simulink model "TruckBenchmark"  (R2023a)
settings: Solver=FixedStepAuto  StartTime=0.0  StopTime=sim_time  FixedStep=control.Ts  MaxStep=1  RelTol=1e-3  EnableMultiTasking=on
StartFcn:
  | tic
StopFcn:
  | simt=toc;
  | fprintf('Simulation time %.3f s\n',simt)
  | TruckBenchmark_Evaluation
values from neighbouring files (symbols this model uses):
  attack_duration = input('Enter the duration of each attack: ')    [RunMe.m]
  attack_freq = input('Enter the desired frequency of attack: ')    [RunMe.m]
  attack_time = input('Enter the time for attack: ')    [RunMe.m]
  attack_type = input('Select the type of Attack (1= Fuzzy, 2=spoofing, 3=Plateau, 4=Replay Attack, 5 = GAttack, 6= C-GAttack, 7= No Attack, 8 = Denial of Service):')    [RunMe.m]
  can_sample_time = 0.001    [runSim.m]
  clutch_pos = TruckBenchmark_Result.find('clutch_pos').Values    [TruckBenchmark_Evaluation.m]
  control =     [TruckBenchmark_Control.mat]
  cruise_profile = input('Select Cruise Profile (Step decrease = 1, Constant 80kph = 2): ')    [RunMe.m]
  curr_gear = TruckBenchmark_Result.find('curr_gear').Values    [TruckBenchmark_Evaluation.m]
  DoS = 0    [RunMe.m]
  gattack_data = interp1(original_time, data, desired_time, 'linear')    [RunMe.m]
  gattack_time = desired_time    [RunMe.m]
  k_slope = TruckBenchmark_Result.find('k_slope').Values    [TruckBenchmark_Evaluation.m]
  lambda = TruckBenchmark_Result.find('lambda').Values    [TruckBenchmark_Evaluation.m]
  model =     [TruckBenchmark_Data.mat]
  n_engine = TruckBenchmark_Result.find('n_engine').Values    [TruckBenchmark_Evaluation.m]
  road = scenario.road    [runSim.m]
  scenario =     [Sodertalje_Norrkoping_Scenario.mat]
  sim_time = input('Enter the total simulation time: ')    [RunMe.m]
  spoofed_value = input('Set the spoofing value:')    [RunMe.m]
  ts = struct('orig_30kph', ts_orig_30kph, 'gen_30kph', ts_gen_30kph, 'orig_40kph', ts_orig_40kph, 'gen_40kph', ts_gen_40kph, 'orig_50kph', ts_orig_50kph, 'gen_50kph', ts_gen_50kph, 'orig_60kph', ts_orig_60kph, 'gen_60kph', ts_gen_60kph,'orig_70kph', ts_orig_70kph, 'gen_70kph', ts_gen_70kph, 'orig_80kph', ts_orig_80kph, 'gen_80kph', ts_gen_80kph, 'orig_90kph', ts_orig_90kph, 'gen_90kph', ts_gen_90kph)    [data_to_mat.m]
  v_vehicle = 0    [RunMe.m]    (also in TruckBenchmark_Evaluation.m = TruckBenchmark_Result.find('v_vehicle').Values)
undefined symbols (not defined in the file or in its folder): canChannel, CCVS, DiscIntNeverNeededParam, dm_airInlet, EGF1, ESSI, ETC2, gcbh, IMT1, n_t, p_inletManifold, r_egr, VD, VDHR, x_distance
libraries: j1939protocollib x25, simulink x5, canlib x2, j1939tllib x2, canmsglib x1, vntj1939tllib x1, slpidlib x1
(part 2 of 4)

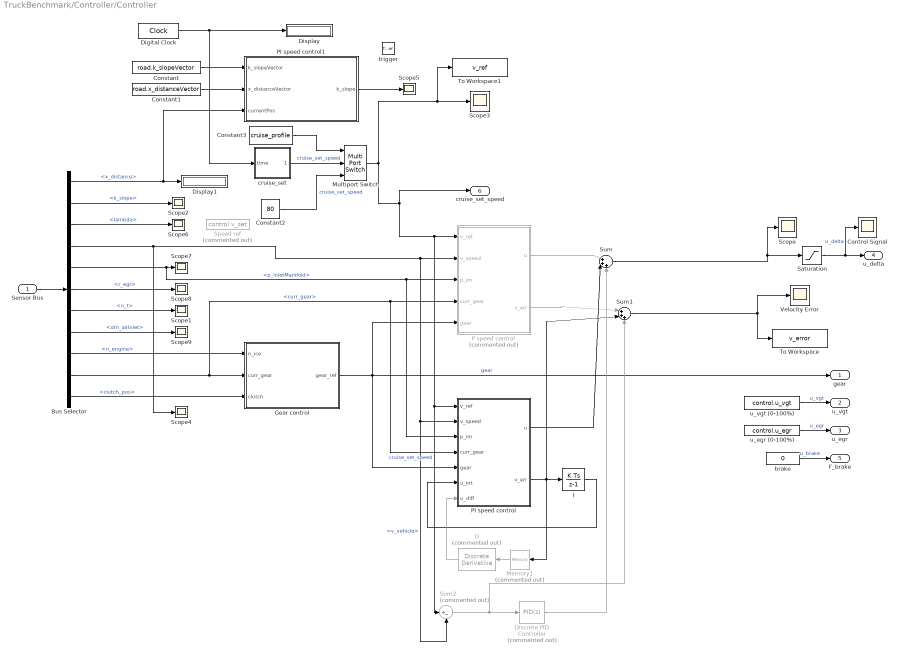
== system TruckBenchmark/Controller/Controller ==
  Sensor Bus : Inport
  trigger : TriggerPort  TriggerType=function-call  VariantControl=(inherit)  PortDimensions=1
  Bus Selector : BusSelector  OutputSignals=x_distance,k_slope,lambda,v_vehicle,p_inletManifold,r_egr,n_t,dm_airInlet,n_engine,curr_gear,clutch_pos
  Constant : Constant  Value=road.k_slopeVector
  Constant1 : Constant  Value=road.x_distanceVector
  Constant2 : Constant  Value=80
  Constant3 : Constant  Value=cruise_profile
  Control Signal : Scope
  D : simulink/Discrete/Discrete Derivative  Commented=on  gainval=1.0  ICPrevScaledInput=0.0  OutMin=[]  OutMax=[]  OutDataType=fixdt(1, 16)  OutScaling=2^-10  DoSatur=off
  Digital Clock : DigitalClock  SampleTime=-1
  Discrete PID Controller : slpidlib/PID Controller  Commented=on  Controller=PID  Form=Parallel  TimeDomain=Discrete-time  UseExternalTs=off  SampleTime=-1  IntegratorMethod=Forward Euler  FilterMethod=Forward Euler  ControllerParametersSource=internal  P=300  I=150  UseKiTs=off  D=0  N=1  UseFilter=on  TunerSelectOption=Transfer Function Based (PID Tuner App)  InitialConditionSource=internal  InitialConditionForIntegrator=0  InitialConditionForFilter=0  DifferentiatorICPrevScaledInput=0  ExternalReset=none  TrackingMode=off  Kt=1  LimitOutput=off  SatLimitsSource=internal  UpperSaturationLimit=inf  LowerSaturationLimit=-inf  LinearizeAsGain=off  AntiWindupMode=none  Kb=1  LimitIntegrator=off  UpperIntegratorSaturationLimit=inf  LowerIntegratorSaturationLimit=-inf  POutMin=[]  POutMax=[]  IOutMin=[]  IOutMax=[]  DOutMin=[]  DOutMax=[]  NOutMin=[]  NOutMax=[]  SumOutMin=[]  SumOutMax=[]  SaturationOutMin=[]  SaturationOutMax=[]  PParamMin=[]  PParamMax=[]  IParamMin=[]  IParamMax=[]  DParamMin=[]  DParamMax=[]  NParamMin=[]  NParamMax=[]  KbParamMin=[]  KbParamMax=[]  KtParamMin=[]  KtParamMax=[]  KbOutMin=[]  KbOutMax=[]  KtOutMin=[]  KtOutMax=[]  IntegratorOutMin=[]  IntegratorOutMax=[]  FilterOutMin=[]  FilterOutMax=[]  SumI1OutMin=[]  SumI1OutMax=[]  SumI2OutMin=[]  SumI2OutMax=[]  SumI3OutMin=[]  SumI3OutMax=[]  SumI4OutMin=[]  SumI4OutMax=[]  SumDOutMin=[]  SumDOutMax=[]  DifferentiatorOutMin=[]  DifferentiatorOutMax=[]  FilterDiffOutCoefMin=[]  FilterDiffOutCoefMax=[]  ReciprocalOutMin=[]  ReciprocalOutMax=[]  SumDenOutMin=[]  SumDenOutMax=[]  SumNumOutMin=[]  SumNumOutMax=[]  DivideOutMin=[]  DivideOutMax=[]  UdiffTsProdOutMin=[]  UdiffTsProdOutMax=[]  NTsProdOutMin=[]  NTsProdOutMax=[]  UintegralTsProdOutMin=[]  UintegralTsProdOutMax=[]  UngainTsProdOutMin=[]  UngainTsProdOutMax=[]  ClampingZeroOutDataTypeStr=Inherit: Inherit via back propagation  ClampingZeroOutMin=[]  ClampingZeroOutMax=[]  FilterDenConstantOutDataTypeStr=Inherit: Inherit via back propagation  FilterDenConstantOutMin=[]  FilterDenConstantOutMax=[]  PCopyOutDataTypeStr=Inherit: Inherit via back propagation  PCopyOutMin=[]  PCopyOutMax=[]  NCopyOutDataTypeStr=Inherit: Inherit via back propagation  NCopyOutMin=[]  NCopyOutMax=[]  IntegratorContinuousStateAttributes=''  IntegratorStateMustResolveToSignalObject=off  IntegratorRTWStateStorageClass=Auto  FilterContinuousStateAttributes=''  FilterStateMustResolveToSignalObject=off  FilterRTWStateStorageClass=Auto  ParallelPVariant=InternalParameters  IdealPVariant=Disabled  IVariant=InternalParameters  DVariant=InternalParameters  IntegratorVariant=Discrete  SatVariant=Disabled  AWVariant=Passthrough  PCopyVariant=Disabled  TRVariant=Disabled  FdbkBlocksVariant=Forward  IdealPFdbkVariant=Disabled  SatFdbkVariant=Disabled  DerivativeFilterVariant=ForwardEulerFilter  NVariant=InternalParameters  NCopyVariant=Disabled  FilterICVariant=InternalICsFilter  IntegratorICVariant=InternalICs  ExternalResetVariant=Disabled  TRSumVariant=Passthrough  SumFdbkVariant=Disabled  SumVariant=Sum_PID  TsampFilterVariant=InternalTs  TsampNgainVariant=Passthrough  TsampIntegralVariant=Disabled_SignalSpec  ExternalSaturationOutDataTypeStr=Inherit: Same as second input
      settings: LibrarySourceBlock=simulink/Discrete/Discrete PID Controller
  Display : Display
  Display1 : Display
  Gear control : MATLAB Function  TreatAsAtomicUnit=on
  I : DiscreteIntegrator  SampleTime=-1  ICPrevOutput=DiscIntNeverNeededParam  ICPrevScaledInput=DiscIntNeverNeededParam
  Memory1 : Memory  Commented=on  InitialCondition=40  InheritSampleTime=on
  Multiport Switch : MultiPortSwitch  Inputs=2  SaturateOnIntegerOverflow=off  InputSameDT=off
  P speed control : MATLAB Function  Commented=on  TreatAsAtomicUnit=on
  PI speed control : MATLAB Function  TreatAsAtomicUnit=on
  PI speed control1 : MATLAB Function  TreatAsAtomicUnit=on
  Saturation : Saturate  UpperLimit=300  LowerLimit=0
  Scope{,1..9} (10 alike) : Scope
  Speed ref : Constant  Commented=on  Value=control.v_set
  Sum : Sum  Inputs=|+++
  Sum1 : Sum  Inputs=|+++
  Sum2 : Sum  Commented=on  Inputs=|+-
  To Workspace : ToWorkspace  VariableName=v_error  SampleTime=-1
  To Workspace1 : ToWorkspace  VariableName=v_ref  SaveFormat=Timeseries  SampleTime=-1
  Velocity Error : Scope
  brake : Constant  Value=0
  cruise_set : MATLAB Function  TreatAsAtomicUnit=on
  u_egr (0-100%) : Constant  Value=control.u_egr
  u_vgt (0-100%) : Constant  Value=control.u_vgt
  gear : Outport  InitialOutput=0
  u_vgt : Outport  Port=2  InitialOutput=0
  u_egr : Outport  Port=3  InitialOutput=0
  u_delta : Outport  Port=4  InitialOutput=0
  F_brake : Outport  Port=5  InitialOutput=0
  cruise_set_speed : Outport  Port=6  InitialOutput=0
  wires:
  Saturation/1 -> Control Signal/1, u_delta/1  "u_delta"
  u_vgt (0-100%)/1 -> u_vgt/1  "u_vgt"
  u_egr (0-100%)/1 -> u_egr/1  "u_egr"
  brake/1 -> F_brake/1  "u_brake"
  Digital Clock/1 -> cruise_set/1(time), Display/1
  Constant/1 -> PI speed control1/1(k_slopeVector)
  Constant1/1 -> PI speed control1/2(x_distanceVector)
  PI speed control1/1(k_slope) -> Scope5/1
  Sensor Bus/1 -> Bus Selector/1
  Bus Selector/5 -> Scope7/1, PI speed control/3(p_im), P speed control/3(p_im)  "<p_inletManifold>"
  Bus Selector/3 -> Scope6/1  "<lambda>"
  Bus Selector/1 -> Display1/1, PI speed control1/3(currentPos)  "<x_distance>"
  Bus Selector/6 -> Scope8/1  "<r_egr>"
  Bus Selector/2 -> Scope2/1  "<k_slope>"
  Bus Selector/8 -> Scope9/1  "<dm_airInlet>"
  Bus Selector/9 -> Gear control/1(n_ice)  "<n_engine>"
  Bus Selector/4 -> Scope4/1, Sum2/2, PI speed control/2(v_speed), P speed control/2(v_speed)  "<v_vehicle>"
  Bus Selector/7 -> Scope1/1  "<n_t>"
  Bus Selector/10 -> Gear control/2(curr_gear), PI speed control/4(curr_gear), P speed control/4(curr_gear)  "<curr_gear>"
  Gear control/1(gear_ref) -> PI speed control/5(gear), gear/1, P speed control/5(gear)  "gear"
  Bus Selector/11 -> Gear control/3(clutch)  "<clutch_pos>"
  Sum1/1 -> To Workspace/1, Velocity Error/1
  Multiport Switch/1 -> cruise_set_speed/1, P speed control/1(v_ref), PI speed control/1(v_ref), Sum2/1, Scope3/1, To Workspace1/1  "cruise_set_speed"
  Sum/1 -> Saturation/1, Scope/1
  P speed control/1(u) -> Sum/1
  PI speed control/1(u) -> Sum/2
  P speed control/2(v_err) -> Sum1/1
  PI speed control/2(v_err) -> I/1, Memory1/1, Sum1/2
  I/1 -> PI speed control/6(u_int)
  Sum2/1 -> Sum1/3, Discrete PID Controller/1
  Discrete PID Controller/1 -> Sum/3
  D/1 -> PI speed control/7(u_diff)
  Memory1/1 -> D/1
  cruise_set/1(cruise_set_speed) -> Multiport Switch/2  "cruise_set_speed"
  Constant2/1 -> Multiport Switch/3  "cruise_set_speed"
  Constant3/1 -> Multiport Switch/1

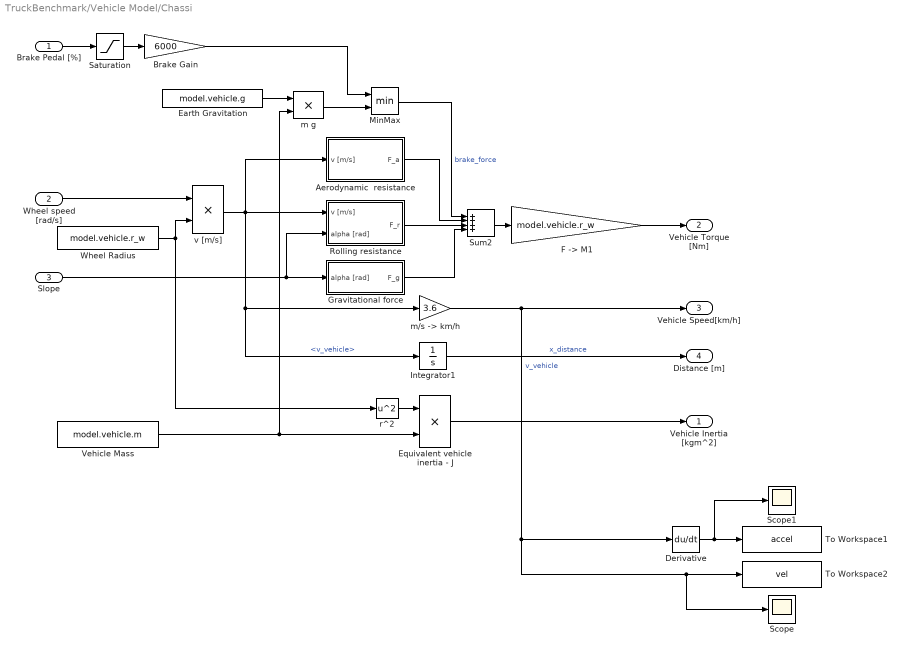
== system TruckBenchmark/Vehicle Model/Chassi ==
  Brake Pedal [%] : Inport
  Wheel speed [rad/s] : Inport  Port=2
  Slope : Inport  Port=3
  Aerodynamic  resistance : Subsystem  mask(Air Drag Subsystem){C_d=model.vehicle.C_d, rho=model.vehicle.rho, Area=model.vehicle.A}
      mask prompts: C_d "C_d - Drag Coefficient  [-]"; rho "rho - Air density [kg/m^3]"; Area "A - Area [m^2]"
      mask help:
      | Calculates the air drag given input vehicle velocity, v, constant values on
      | cross section area, A, drag coefficient, C_d, and air density, rho.
      |
      | Implemented Equation:
      | F_a=0.5 rho C_d A v^2
  Brake Gain : Gain  Gain=6000  SaturateOnIntegerOverflow=on  OutDataTypeStr=Inherit: Same as input  ParamDataTypeStr=Inherit: Same as input
  Derivative : Derivative
  Earth Gravitation : Constant  Value=model.vehicle.g
  Equivalent vehicle inertia - J : Product  SaturateOnIntegerOverflow=on  OutDataTypeStr=Inherit: Same as first input
  "F -> M1" : Gain  Gain=model.vehicle.r_w  SaturateOnIntegerOverflow=on  OutDataTypeStr=Inherit: Same as input  ParamDataTypeStr=Inherit: Same as input
  Gravitational force : Subsystem  mask(Rolling resistance subsystem){m=model.vehicle.m, g=model.vehicle.g}
      mask prompts: m "m - Vehicle mass"; g "g - Gravity of Earth"
      mask help:
      | Calculates the gravitational force given the road slope, alpha, as input
      | and constants for vehicle mass, m, and earth gravitation.
      |
      | Model Equation:
      | F_r = m g sin(alpha)
  Integrator1 : Integrator  LimitOutput=on  LowerSaturationLimit=0
  MinMax : MinMax  Inputs=2
  Rolling resistance : Subsystem  mask(Rolling resistance subsystem){m=model.vehicle.m, g=model.vehicle.g, c_r0=model.vehicle.c_r0, c_r1=model.vehicle.c_r1}
      mask prompts: m "m - Vehicle massm"; g "g - Gravity of Earth"; c_r0 "c_r0 - Rolling resistance coeff"; c_r1 "c_r1 - Rolling resistanc coeff"
      mask help:
      | Calculates the rolling resistance force of a vehicle of mass, m, at
      | vehicle speed, v.
      |
      | Model Equation:
      | F_r = m g cos(alpha) (c_r0 + c_r1 v)
  Saturation : Saturate  UpperLimit=100  LowerLimit=0
  Scope : Scope
  Scope1 : Scope
  Sum2 : Sum  Inputs=++++  SaturateOnIntegerOverflow=on
  To Workspace1 : ToWorkspace  VariableName=accel  SampleTime=-1
  To Workspace2 : ToWorkspace  VariableName=vel  SampleTime=-1
  Vehicle Mass : Constant  Value=model.vehicle.m
  Wheel Radius : Constant  Value=model.vehicle.r_w
  m g : Product  SaturateOnIntegerOverflow=on  OutDataTypeStr=Inherit: Same as first input
  "m/s -> km/h" : Gain  Gain=3.6  SaturateOnIntegerOverflow=on  OutDataTypeStr=Inherit: Same as input  ParamDataTypeStr=Inherit: Same as input
  r^2 : Math  Operator=square  SignedPower=on
  v [m/s] : Product  SaturateOnIntegerOverflow=on  OutDataTypeStr=Inherit: Same as first input
  Vehicle Inertia [kgm^2] : Outport  VectorParamsAs1DForOutWhenUnconnected=off
  Vehicle Torque [Nm] : Outport  Port=2  VectorParamsAs1DForOutWhenUnconnected=off
  Vehicle Speed[km/h] : Outport  Port=3  VectorParamsAs1DForOutWhenUnconnected=off
  Distance [m] : Outport  Port=4  VectorParamsAs1DForOutWhenUnconnected=off
  wires:
  Brake Pedal [%]/1 -> Saturation/1
  Wheel Radius/1 -> r^2/1, v [m/s]/2
  "m/s -> km/h"/1 -> Scope/1, To Workspace2/1, Derivative/1, Vehicle Speed[km/h]/1  "v_vehicle"
  "F -> M1"/1 -> Vehicle Torque [Nm]/1
  Equivalent vehicle inertia - J/1 -> Vehicle Inertia [kgm^2]/1
  Wheel speed [rad/s]/1 -> v [m/s]/1
  Sum2/1 -> "F -> M1"/1
  Slope/1 -> Rolling resistance/2(alpha [rad]), Gravitational force/1(alpha [rad])
  r^2/1 -> Equivalent vehicle inertia - J/1
  Vehicle Mass/1 -> m g/2, Equivalent vehicle inertia - J/2
  Integrator1/1 -> Distance [m]/1  "x_distance"
  Brake Gain/1 -> MinMax/1
  m g/1 -> MinMax/2
  Earth Gravitation/1 -> m g/1
  Saturation/1 -> Brake Gain/1
  MinMax/1 -> Sum2/1  "brake_force"
  Aerodynamic  resistance/1(F_a) -> Sum2/2
  Rolling resistance/1(F_r) -> Sum2/3
  Gravitational force/1(F_g) -> Sum2/4
  v [m/s]/1 -> Aerodynamic  resistance/1(v [m/s]), Rolling resistance/1(v [m/s]), Integrator1/1, "m/s -> km/h"/1  "<v_vehicle>"
  Derivative/1 -> Scope1/1, To Workspace1/1

== system TruckBenchmark/Vehicle Model/Clutch and Transmission ==
  M_e [Nm] : Inport
  Gear : Inport  Port=2
  Clutch Pos [0...1] : Inport  Port=3
  J_e : Inport  Port=4
  M_veh [Nm] : Inport  Port=5
  J_veh : Inport  Port=6
  Clutch Transfer : Subsystem
  Engine Dynamics : Subsystem
  Final Drive gear ratio : Gain  Gain=model.transmission.i_f
  Gear box gear ratios : Lookup  InputValues=model.transmission.r_gearNumbers  Table=model.transmission.r_gearRatios
  Mux : Mux  Inputs=5
  Speed Difference Clutch Limits : Subsystem
  Vehicle Dynamics : Subsystem
  w_e [rad/s] : Outport  VectorParamsAs1DForOutWhenUnconnected=off
  w_wheel [rad/s] : Outport  Port=2  VectorParamsAs1DForOutWhenUnconnected=off
  wires:
  M_e [Nm]/1 -> Engine Dynamics/2(Tq_e), Mux/1
  J_e/1 -> Engine Dynamics/3(J_e), Mux/2
  Gear/1 -> Gear box gear ratios/1
  M_veh [Nm]/1 -> Vehicle Dynamics/2(Tq_veh), Mux/3
  J_veh/1 -> Vehicle Dynamics/3(J_v), Mux/4
  Clutch Pos [0...1]/1 -> Speed Difference Clutch Limits/1(Clutch [0...1])
  Engine Dynamics/1(w_e) -> w_e [rad/s]/1, Speed Difference Clutch Limits/2(w_e)  "omega_e"
  Clutch Transfer/1(M_c) -> Vehicle Dynamics/1(Tq_c), Engine Dynamics/1(Tq_c)  "M_c"
  Mux/1 -> Clutch Transfer/3(Insignals)
  Speed Difference Clutch Limits/1(Clutch Locked) -> Clutch Transfer/2(Clutch Locked)  "cl_lock"
  Speed Difference Clutch Limits/2(M_c_max) -> Clutch Transfer/1(Tq_c_max)  "M_c_max"
  Vehicle Dynamics/1(w_wheel) -> w_wheel [rad/s]/1, Speed Difference Clutch Limits/3(w_wheel)  "omega_w"
  Gear box gear ratios/1 -> Final Drive gear ratio/1
  Final Drive gear ratio/1 -> Speed Difference Clutch Limits/4(Gear ratio), Vehicle Dynamics/4(Gear ratio), Mux/5

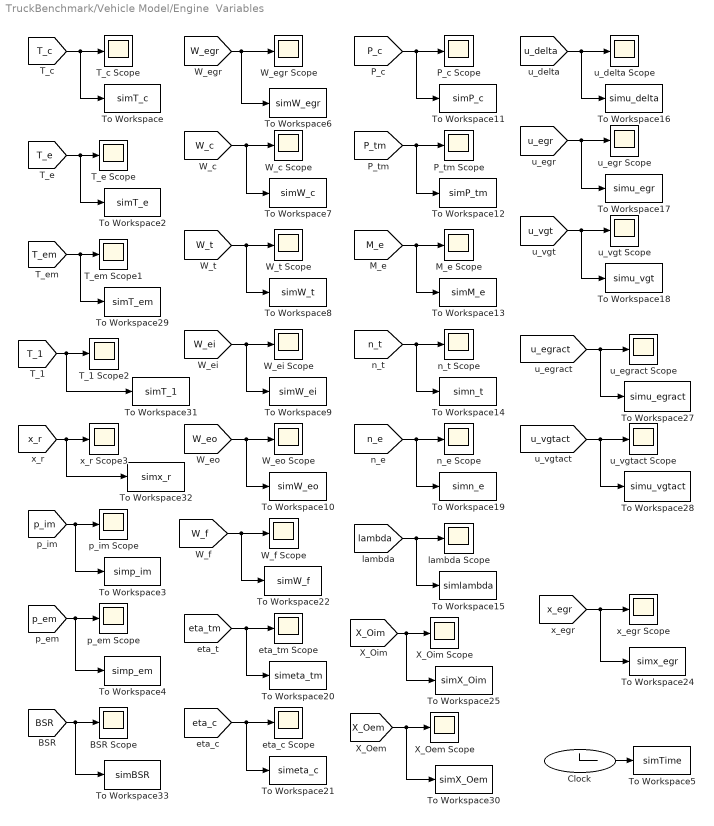
== system TruckBenchmark/Vehicle Model/Engine  Variables ==
  BSR Scope : Scope
  Clock : Clock
  M_e Scope : Scope
  P_c Scope : Scope
  P_tm Scope : Scope
  T_1 Scope2 : Scope
  T_c Scope : Scope
  T_e Scope : Scope
  T_em Scope1 : Scope
  To Workspace : ToWorkspace  VariableName=simT_c  SampleTime=-1
  To Workspace10 : ToWorkspace  VariableName=simW_eo  SampleTime=-1
  To Workspace11 : ToWorkspace  VariableName=simP_c  SampleTime=-1
  To Workspace12 : ToWorkspace  VariableName=simP_tm  SampleTime=-1
  To Workspace13 : ToWorkspace  VariableName=simM_e  SampleTime=-1
  To Workspace14 : ToWorkspace  VariableName=simn_t  SampleTime=-1
  To Workspace15 : ToWorkspace  VariableName=simlambda  SampleTime=-1
  To Workspace16 : ToWorkspace  VariableName=simu_delta  SampleTime=-1
  To Workspace17 : ToWorkspace  VariableName=simu_egr  SampleTime=-1
  To Workspace18 : ToWorkspace  VariableName=simu_vgt  SampleTime=-1
  To Workspace19 : ToWorkspace  VariableName=simn_e  SampleTime=-1
  To Workspace2 : ToWorkspace  VariableName=simT_e  SampleTime=-1
  To Workspace20 : ToWorkspace  VariableName=simeta_tm  SampleTime=-1
  To Workspace21 : ToWorkspace  VariableName=simeta_c  SampleTime=-1
  To Workspace22 : ToWorkspace  VariableName=simW_f  SampleTime=-1
  To Workspace24 : ToWorkspace  VariableName=simx_egr  SampleTime=-1
  To Workspace25 : ToWorkspace  VariableName=simX_Oim  SampleTime=-1
  To Workspace27 : ToWorkspace  VariableName=simu_egract  SampleTime=-1
  To Workspace28 : ToWorkspace  VariableName=simu_vgtact  SampleTime=-1
  To Workspace29 : ToWorkspace  VariableName=simT_em  SampleTime=-1
  To Workspace3 : ToWorkspace  VariableName=simp_im  SampleTime=-1
  To Workspace30 : ToWorkspace  VariableName=simX_Oem  SampleTime=-1
  To Workspace31 : ToWorkspace  VariableName=simT_1  SampleTime=-1
  To Workspace32 : ToWorkspace  VariableName=simx_r  SampleTime=-1
  To Workspace33 : ToWorkspace  VariableName=simBSR  SampleTime=-1
  To Workspace4 : ToWorkspace  VariableName=simp_em  SampleTime=-1
  To Workspace5 : ToWorkspace  VariableName=simTime  SampleTime=-1
  To Workspace6 : ToWorkspace  VariableName=simW_egr  SampleTime=-1
  To Workspace7 : ToWorkspace  VariableName=simW_c  SampleTime=-1
  To Workspace8 : ToWorkspace  VariableName=simW_t  SampleTime=-1
  To Workspace9 : ToWorkspace  VariableName=simW_ei  SampleTime=-1
  W_c Scope : Scope
  W_egr Scope : Scope
  W_ei Scope : Scope
  W_eo Scope : Scope
  W_f Scope : Scope
  W_t Scope : Scope
  X_Oem Scope : Scope
  X_Oim Scope : Scope
  eta_c Scope : Scope
  eta_tm Scope : Scope
  lambda Scope : Scope
  n_e Scope : Scope
  n_t Scope : Scope
  p_em Scope : Scope
  p_im Scope : Scope
  u_delta Scope : Scope
  u_egr Scope : Scope
  u_egract Scope : Scope
  u_vgt Scope : Scope
  u_vgtact Scope : Scope
  x_egr Scope : Scope
  x_r Scope3 : Scope
  wires:
  [u_vgtact] -> To Workspace28/1, u_vgtact Scope/1
  [u_egract] -> u_egract Scope/1, To Workspace27/1
  [x_egr] -> x_egr Scope/1, To Workspace24/1
  [W_f] -> W_f Scope/1, To Workspace22/1
  [eta_c] -> To Workspace21/1, eta_c Scope/1
  [eta_tm] -> eta_tm Scope/1, To Workspace20/1
  [n_e] -> n_e Scope/1, To Workspace19/1
  [u_vgt] -> u_vgt Scope/1, To Workspace18/1
  [u_egr] -> To Workspace17/1, u_egr Scope/1
  [u_delta] -> u_delta Scope/1, To Workspace16/1
  Clock/1 -> To Workspace5/1
  [lambda] -> To Workspace15/1, lambda Scope/1
  [M_e] -> To Workspace13/1, M_e Scope/1
  [W_eo] -> To Workspace10/1, W_eo Scope/1
  [P_tm] -> To Workspace12/1, P_tm Scope/1
  [P_c] -> To Workspace11/1, P_c Scope/1
  [W_ei] -> To Workspace9/1, W_ei Scope/1
  [W_t] -> To Workspace8/1, W_t Scope/1
  [W_c] -> To Workspace7/1, W_c Scope/1
  [W_egr] -> To Workspace6/1, W_egr Scope/1
  [n_t] -> To Workspace14/1, n_t Scope/1
  [p_em] -> To Workspace4/1, p_em Scope/1
  [p_im] -> To Workspace3/1, p_im Scope/1
  [T_e] -> To Workspace2/1, T_e Scope/1
  [T_c] -> To Workspace/1, T_c Scope/1
  [T_em] -> T_em Scope1/1, To Workspace29/1
  [X_Oem] -> X_Oem Scope/1, To Workspace30/1
  [X_Oim] -> X_Oim Scope/1, To Workspace25/1
  [T_1] -> T_1 Scope2/1, To Workspace31/1
  [x_r] -> x_r Scope3/1, To Workspace32/1
  [BSR] -> BSR Scope/1, To Workspace33/1

== system TruckBenchmark/Vehicle Model/ICE ==
  u_vgt : Inport
  u_egr : Inport  Port=2
  u_delta : Inport  Port=3
  n_e : Inport  Port=4
  Cylinder : Subsystem  mask{n_cyl=model.engine.n_cyl, AFs=model.engine.AFs, q_HV=model.engine.q_HV, V_d=model.engine.V_d, r_c=model.engine.r_c}
  EGR-system : Subsystem  mask{PI_egropt=model.engine.PI_egropt, c_egr=model.engine.c_egr, uInit_egr=model.engine.uInit_egr, A_egrmax=model.engine.A_egrmax}
  Exhaust Manifold : Subsystem  mask{p_em_Init=model.engine.p_em_Init, V_em=model.engine.V_em}
  Inlet Manifold temp : Constant  Value=T_im
  Intake Manifold : Subsystem  mask{p_im_Init=model.engine.p_im_Init, V_im=model.engine.V_im}
  Turbo : Subsystem
  M_e : Outport  VectorParamsAs1DForOutWhenUnconnected=off
  m_fuelTot : Outport  Port=2  VectorParamsAs1DForOutWhenUnconnected=off
  r_lambdaOut : Outport  Port=3  VectorParamsAs1DForOutWhenUnconnected=off
  p_inletManifold : Outport  Port=4  VectorParamsAs1DForOutWhenUnconnected=off
  r_egr : Outport  Port=5  VectorParamsAs1DForOutWhenUnconnected=off
  W_c : Outport  Port=6  VectorParamsAs1DForOutWhenUnconnected=off
  n_t : Outport  Port=7  VectorParamsAs1DForOutWhenUnconnected=off
  tag scope: T_c=global
  wires:
  Exhaust Manifold/2(X_Oem) -> Intake Manifold/5(X_Oem)
  Cylinder/4(X_Oe) -> Exhaust Manifold/5(X_Oe)
  Intake Manifold/2(X_Oim) -> Cylinder/3(X_Oim)
  u_delta/1 -> Cylinder/5(u_delta)
  n_e/1 -> Cylinder/4(n_e)
  Turbo/2(T_c) -> [T_c]
  u_vgt/1 -> Turbo/4(u_vgt)
  u_egr/1 -> EGR-system/4(u_egr)
  Cylinder/3(T_em) -> EGR-system/2(T_em), Exhaust Manifold/4(T_em), Turbo/3(T_em)
  Cylinder/1(W_ei) -> Intake Manifold/3(W_ei)
  Inlet Manifold temp/1 -> Intake Manifold/4(T_im), Cylinder/6(T_im)
  Turbo/1(W_c) -> Intake Manifold/1(W_c), W_c/1
  EGR-system/1(W_egr) -> Intake Manifold/2(W_egr), Exhaust Manifold/3(W_egr)
  Turbo/3(W_t) -> Exhaust Manifold/2(W_t)
  Cylinder/2(W_eo) -> Exhaust Manifold/1(W_eo)
  Exhaust Manifold/1(p_em) -> EGR-system/3(p_em), Cylinder/2(p_em), Turbo/2(p_em)
  Intake Manifold/1(p_im) -> p_inletManifold/1, Turbo/1(p_im), Cylinder/1(p_im), EGR-system/1(p_im)  "p_inletManifold"
  Cylinder/5(M_e) -> M_e/1
  Cylinder/6(m_fuelTot) -> m_fuelTot/1
  Cylinder/7(r_lambdaOut) -> r_lambdaOut/1
  Intake Manifold/3(r_egr) -> r_egr/1
  Turbo/4(n_t) -> n_t/1

== system TruckBenchmark/Vehicle Model/Road Slope Data ==
  x_distance : Inport
  v [km/h] : Inport  Port=2
  1-D Lookup Table : Lookup_n-D  NumberOfTableDimensions=1  BreakpointsForDimension1=road.x_distanceVector  BeginIndexSearchUsingPreviousIndexResult=on  Table=road.k_slopeVector  InterpMethod=Cubic spline  RndMeth=Simplest
  Constant : Constant  Value=road.x_distanceVector(end)
  Integrator : Integrator  InitialCondition=scenario.h_0  LowerSaturationLimit=0
  Relational Operator : RelationalOperator  OutDataTypeStr=boolean  InputSameDT=off
  Scope1 : Scope
  Scope2 : Scope
  Stop Simulation : Stop
  Trigonometric Function : Trigonometry
  h dot : Product  Inputs=**  InputSameDT=on  SaturateOnIntegerOverflow=on  OutDataTypeStr=Inherit: Same as first input
  "km/h -> m/s " : Gain  Gain=1/3.6  SaturateOnIntegerOverflow=on  OutDataTypeStr=Inherit: Same as input  ParamDataTypeStr=Inherit: Same as input
  altitude [m] : Outport  VectorParamsAs1DForOutWhenUnconnected=off
  slope [rad] : Outport  Port=2  VectorParamsAs1DForOutWhenUnconnected=off
  wires:
  x_distance/1 -> Relational Operator/1, 1-D Lookup Table/1, Scope2/1
  1-D Lookup Table/1 -> Trigonometric Function/1, slope [rad]/1, Scope1/1  "k_slope"
  Constant/1 -> Relational Operator/2
  Relational Operator/1 -> Stop Simulation/1
  v [km/h]/1 -> "km/h -> m/s "/1
  Trigonometric Function/1 -> h dot/1
  "km/h -> m/s "/1 -> h dot/2
  h dot/1 -> Integrator/1
  Integrator/1 -> altitude [m]/1  "altitude"

== system TruckBenchmark/Controller/CAN TX//RX/ Periodic Trigger1 ==
  Relational Operator : RelationalOperator  OutDataTypeStr=boolean  InputSameDT=off
  Repetition Interval : Constant  Value=repetitionInterval
  Timer : Subsystem
  Unit Delay : UnitDelay  InitialCondition=1  SampleTime=-1  HasFrameUpgradeWarning=on
  Trigger : Outport  OutputWhenDisabled=reset  InitialOutput=0  VectorParamsAs1DForOutWhenUnconnected=off
  wires:
  Timer/1(Timer Value (ms)) -> Relational Operator/1
  Repetition Interval/1 -> Relational Operator/2
  Unit Delay/1 -> Timer/1(Reset)
  Relational Operator/1 -> Trigger/1, Unit Delay/1  "Trigger Pulse"

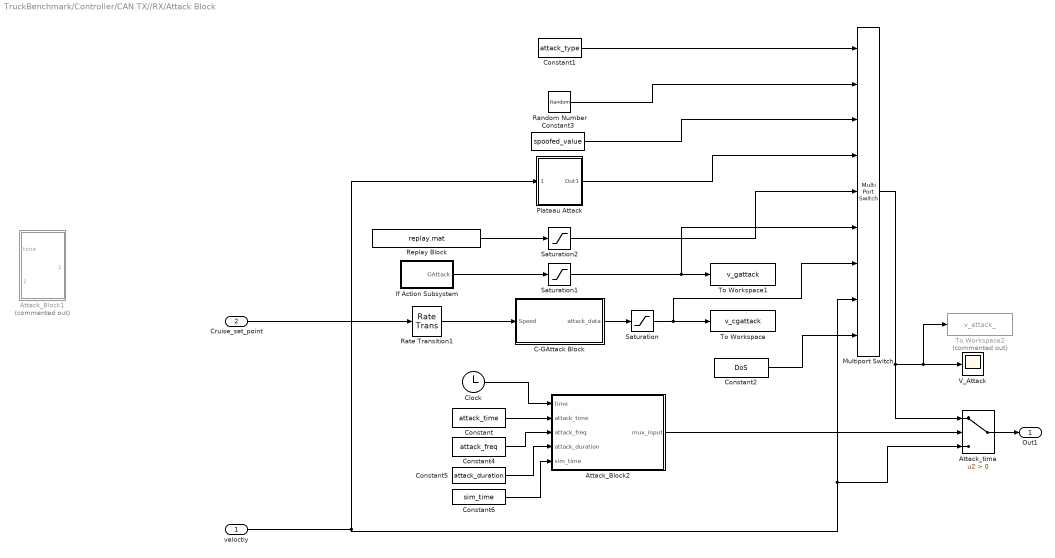
== system TruckBenchmark/Controller/CAN TX//RX/Attack Block ==
  veloctiy : Inport
  Cruise_set_point : Inport  Port=2
  Attack_Block1 : MATLAB Function  Commented=on  TreatAsAtomicUnit=on
  Attack_Block2 : MATLAB Function  TreatAsAtomicUnit=on
  Attack_time : Switch  Criteria=u2 > Threshold  SaturateOnIntegerOverflow=off  InputSameDT=off
  C-GAttack Block : Subsystem
  Clock : Clock
  Constant : Constant  Value=attack_time
  Constant1 : Constant  Value=attack_type
  Constant2 : Constant  Value=DoS
  Constant3 : Constant  Value=spoofed_value
  Constant4 : Constant  Value=attack_freq
  Constant5 : Constant  Value=attack_duration
  Constant6 : Constant  Value=sim_time
  If Action Subsystem : Subsystem  TreatAsAtomicUnit=on
  Multiport Switch : MultiPortSwitch  Inputs=8  SaturateOnIntegerOverflow=off  InputSameDT=off
  Plateau Attack : Subsystem
  Random Number : RandomNumber  Mean=v_vehicle  Variance=255  Seed=10  SampleTime=can_sample_time
  Rate Transition1 : RateTransition
  Replay Block : FromFile  FileName=replay.mat  OutDataTypeStr=double  SampleTime=can_sample_time
  Saturation : Saturate  UpperLimit=inf  LowerLimit=0
  Saturation1 : Saturate  UpperLimit=inf  LowerLimit=0
  Saturation2 : Saturate  UpperLimit=inf  LowerLimit=0
  To Workspace : ToWorkspace  VariableName=v_cgattack  SaveFormat=Timeseries  SampleTime=-1
  To Workspace1 : ToWorkspace  VariableName=v_gattack  SaveFormat=Timeseries  SampleTime=-1
  To Workspace2 : ToWorkspace  Commented=on  VariableName=v_attack_  SaveFormat=Timeseries  SampleTime=-1
  V_Attack : Scope
  Out1 : Outport
  wires:
  Rate Transition1/1 -> C-GAttack Block/1(Speed)
  If Action Subsystem/1(GAttack) -> Saturation1/1
  C-GAttack Block/1(attack_data) -> Saturation/1
  Saturation1/1 -> Multiport Switch/6, To Workspace1/1
  Saturation/1 -> Multiport Switch/7, To Workspace/1
  Constant1/1 -> Multiport Switch/1
  Attack_Block2/1(mux_input) -> Attack_time/2
  Clock/1 -> Attack_Block2/1(time)
  Constant/1 -> Attack_Block2/2(attack_time)
  Multiport Switch/1 -> Attack_time/1, To Workspace2/1, V_Attack/1
  Saturation2/1 -> Multiport Switch/5
  Replay Block/1 -> Saturation2/1
  Cruise_set_point/1 -> Rate Transition1/1
  Random Number/1 -> Multiport Switch/2
  Constant3/1 -> Multiport Switch/3
  veloctiy/1 -> Multiport Switch/8, Attack_time/3, Plateau Attack/1(v_vehicle)
  Plateau Attack/1(Out1) -> Multiport Switch/4
  Attack_time/1 -> Out1/1
  Constant2/1 -> Multiport Switch/9
  Constant4/1 -> Attack_Block2/3(attack_freq)
  Constant5/1 -> Attack_Block2/4(attack_duration)
  Constant6/1 -> Attack_Block2/5(sim_time)

== system TruckBenchmark/Controller/CAN TX//RX/CAN Rx 65265 (Velocity, Clutch Pos) ==
  note: Copyright 2015-2021 The MathWorks, Inc.
  J1939 Receive2 : j1939protocollib/J1939 Receive  Priority=-1  ConfigName=Config1  NodeName=Engine1  PGList=CCVS(65265)  PGName=CCVS  MsgLength=8  SignalInfo=BrakeSwitch$28$2$1$2$1$0$1$0$0$3$$597$#ClutchSwitch$30$2$1$2$1$0$1$0$0$3$$598$#CruiseCtrlAccelerateSwitch$38$2$1$2$1$0$1$0$0$3$$602$#CruiseCtrlActive$24$2$1$2$1$0$1$0$0$3$$595$#CruiseCtrlCoastSwitch$34$2$1$2$1$0$1$0$0$3$$600$#CruiseCtrlEnableSwitch$26$2$1$2$1$0$1$0$0$3$$596$#CruiseCtrlPauseSwitch$4$2$1$2$1$0$1$0$0$3$$1633$#CruiseCtrlResumeSwitch$36$2$1$2$1$0$1$0$0$3$$601$#CruiseCtrlSetSpeed$40$8$1$2$1$0$1$0$0$250$km/h$86$#CruiseCtrlSetSwitch$32$2$1$2$1$0$1$0$0$3$$599$#CruiseCtrlStates$53$3$1$2$1$0$1$0$0$7$$527$#EngIdleDecrementSwitch$58$2$1$2$1$0$1$0$0$3$$967$#EngIdleIncrementSwitch$56$2$1$2$1$0$1$0$0$3$$968$#EngShutdownOverrideSwitch$62$2$1$2$1$0$1$0$0$3$$1237$#EngTestModeSwitch$60$2$1$2$1$0$1$0$0$3$$966$#PTOGovernorState$48$5$1$2$1$0$1$0$0$31$$976$#ParkBrakeReleaseInhibitRq$6$2$1$2$1$0$1$0$0$3$$3807$#ParkingBrakeSwitch$2$2$1$2$1$0$1$0$0$3$$70$#TwoSpeedAxleSwitch$0$2$1$2$1$0$1$0$0$3$$69$#WheelBasedVehicleSpeed$8$16$1$2$1$0$3.906250e-03$0$0$2.509960e+02$km/h$84$#  NSignals=20  StartBits=str2num('[double(28);double(30);double(38);double(24);double(34);double(26);double(4);double(36);double(40);double(32);double(53);double(58);double(56);double(62);double(60);double(48);double(6);double(2);double(0);double(8)]')  SignalSizes=str2num('[double(2),double(2),double(2),double(2),double(2),double(2),double(2),double(2),double(8),double(2),double(3),double(2),double(2),double(2),double(2),double(5),double(2),double(2),double(2),double(16)]')  ByteOrders=str2num('[int32(1);int32(1);int32(1);int32(1);int32(1);int32(1);int32(1);int32(1);int32(1);int32(1);int32(1);int32(1);int32(1);int32(1);int32(1);int32(1);int32(1);int32(1);int32(1);int32(1)]')  DataTypes=str2num('[int32(2);int32(2);int32(2);int32(2);int32(2);int32(2);int32(2);int32(2);int32(2);int32(2);int32(2);int32(2);int32(2);int32(2);int32(2);int32(2);int32(2);int32(2);int32(2);int32(2)]')  MultiplexTypes=str2num('[int32(1);int32(1);int32(1);int32(1);int32(1);int32(1);int32(1);int32(1);int32(1);int32(1);int32(1);int32(1);int32(1);int32(1);int32(1);int32(1);int32(1);int32(1);int32(1);int32(1)]')  MultiplexValues=str2num('[double(0);double(0);double(0);double(0);double(0);double(0);double(0);double(0);double(0);double(0);double(0);double(0);double(0);double(0);double(0);double(0);double(0);double(0);double(0);double(0)]')  Factors=str2num('[double(1);double(1);double(1);double(1);double(1);double(1);double(1);double(1);double(1);double(1);double(1);double(1);double(1);double(1);double(1);double(1);double(1);double(1);double(1);double(3.906250e-03)]')  Offsets=str2num('[double(0);double(0);double(0);double(0);double(0);double(0);double(0);double(0);double(0);double(0);double(0);double(0);double(0);double(0);double(0);double(0);double(0);double(0);double(0);double(0)]')  Minimums=str2num('[double(0);double(0);double(0);double(0);double(0);double(0);double(0);double(0);double(0);double(0);double(0);double(0);double(0);double(0);double(0);double(0);double(0);double(0);double(0);double(0)]')  Maximums=str2num('[double(3);double(3);double(3);double(3);double(3);double(3);double(3);double(3);double(250);double(3);double(7);double(3);double(3);double(3);double(3);double(31);double(3);double(3);double(3);double(2.509960e+02)]')  Units=0  SPN=str2num('[double(597);double(598);double(602);double(595);double(600);double(596);double(1633);double(601);double(86);double(599);double(527);double(967);double(968);double(1237);double(966);double(976);double(3807);double(70);double(69);double(84)]')  Comment=0  SrcAddrFilter=Allow all  SrcAddress=255  DestAddrFilter=1  outputNew=off  SampleTime=0.54e-3  ApplyMinMax=off
  Signals3 : Scope  NumInputPorts=4
  Terminator{1,17..31} (16 alike) : Terminator
  rx Vehicle Velocity : Outport
  rx Clutch Pos : Outport  Port=2
  wires:
  J1939 Receive2/17 -> Terminator26/1
  J1939 Receive2/3 -> Terminator24/1
  J1939 Receive2/10 -> Terminator18/1
  J1939 Receive2/5 -> Terminator23/1
  J1939 Receive2/14 -> Terminator28/1
  J1939 Receive2/20 -> Signals3/4, rx Vehicle Velocity/1
  J1939 Receive2/4 -> Terminator19/1
  J1939 Receive2/19 -> Terminator17/1
  J1939 Receive2/15 -> Terminator27/1
  J1939 Receive2/11 -> Terminator31/1
  J1939 Receive2/8 -> Terminator20/1
  J1939 Receive2/13 -> Terminator29/1
  J1939 Receive2/6 -> Terminator22/1
  J1939 Receive2/9 -> Signals3/3
  J1939 Receive2/1 -> Terminator1/1
  J1939 Receive2/12 -> Terminator30/1
  J1939 Receive2/16 -> Signals3/1
  J1939 Receive2/7 -> Terminator21/1
  J1939 Receive2/18 -> Terminator25/1
  J1939 Receive2/2 -> rx Clutch Pos/1, Signals3/2

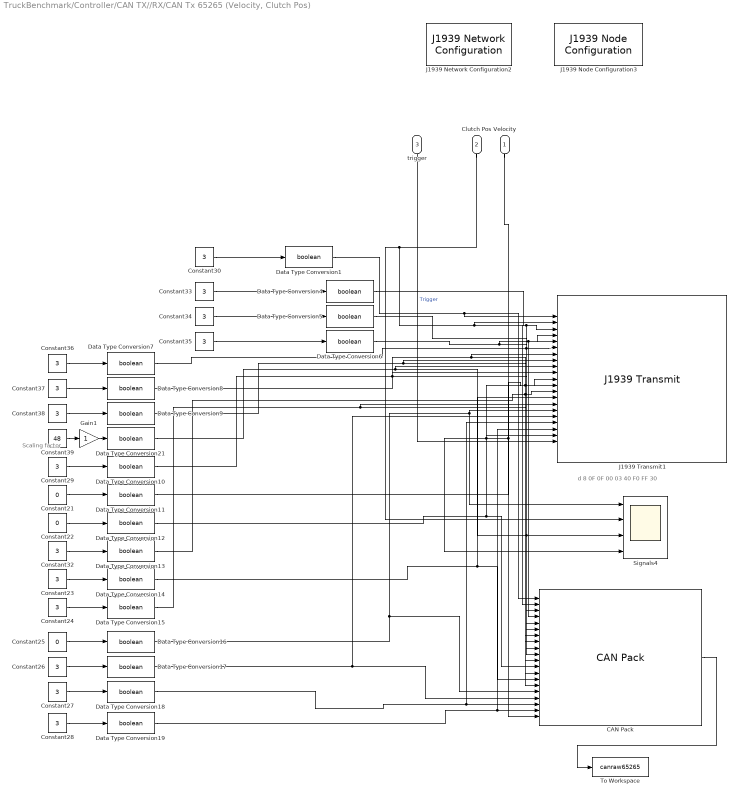
== system TruckBenchmark/Controller/CAN TX//RX/CAN Tx 65265 (Velocity, Clutch Pos) ==
  note: Scaling factor
  note: d 8 0F 0F 00 03 40 F0 FF 30
  Velocity : Inport
  Clutch Pos : Inport  Port=2
  trigger : Inport  Port=3
  CAN Pack : canmsglib/CAN Pack  CANdbFile=C:\Users\qazim\OneDrive - The Ohio State University\Application for Fellowship\.Project\SDCS\J1939 Standards\j1939.dbc  MsgList=CCVS  MsgName=CCVS  MsgIDType=Extended (29-bit identifier)  MsgIdentifier=419361278  MsgLength=8  Remote=off  ApplyMinMax=off  BusOutput=on  SignalInfo={'BrakeSwitch','28','2','LE','unsigned','Standard','0','1','0','0','3';'ClutchSwitch','30','2','LE','unsigned','Standard','0','1','0','0','3';'CruiseCtrlAccelerateSwitch','38','2','LE','unsigned','Standard','0','1','0','0','3';'CruiseCtrlActive','24','2','LE','unsigned','Standard','0','1','0','0','3';'CruiseCtrlCoastSwitch','34','2','LE','unsigned','Standard','0','1','0','0','3';'CruiseCtrlEnableSwitch','26','2','LE','unsigned','Standard','0','1','0','0','3';'CruiseCtrlPauseSwitch','4','2','LE','unsigned','Standard','0','1','0','0','3';'CruiseCtrlResumeSwitch','36','2','LE','unsigned','Standard','0','1','0','0','3';'CruiseCtrlSetSpeed','40','8','LE','unsigned','Standard','0','1','0','0','250';'CruiseCtrlSetSwitch','32','2','LE','unsigned','Standard','0','1','0','0','3';'CruiseCtrlStates','53','3','LE','unsigned','Standard','0','1','0','0','7';'EngIdleDecrementSwitch','58','2','LE','unsigned','Standard','0','1','0','0','3';'EngIdleIncrementSwitch','56','2','LE','unsigned','Standard','0','1','0','0','3';'EngShutdownOverrideSwitch','62','2','LE','unsigned','Standard','0','1','0','0','3';'EngTestModeSwitch','60','2','LE','unsigned','Standard','0','1','0','0','3';'PTOGovernorState','48','5','LE','unsigned','Standard','0','1','0','0','31';'ParkBrakeReleaseInhibitRq','6','2','LE','unsigned','Standard','0','1','0','0','3';'ParkingBrakeSwitch','2','2','LE','unsigned','Standard','0','1','0','0','3';'TwoSpeedAxleSwitch','0','2','LE','unsigned','Standard','0','1','0','0','3';'WheelBasedVehicleSpeed','8','16','LE','unsigned','Standard','0','0.0039062','0','0','250.996'}
      settings: LibrarySourceBlock=canlib/CAN Pack  DataFormat=CANdb specified signals
  Constant21 : Constant  Value=0
  Constant22 : Constant  Value=0
  Constant{23..24,26..30,32..38} (14 alike) : Constant  Value=3
  Constant25 : Constant  Value=0
  Constant39 : Constant  Value=48
  Data Type Conversion{1,4..19,21} (18 alike) : DataTypeConversion  OutDataTypeStr=boolean  SaturateOnIntegerOverflow=off  RndMeth=Floor
  Gain1 : Gain
  J1939 Network Configuration2 : j1939protocollib/J1939 Network Configuration  Priority=-3  ConfigName=Config3  DbFile=C:\Users\qazim\OneDrive - The Ohio State University\Application for Fellowship\.Project\SDCS\Generative AI\Truck Simulink Model\TruckBenchmark_v1.2\TruckBenchmark\j1939.dbc  PrevDbFile=C:\Users\qazim\OneDrive - The Ohio State University\Application for Fellowship\.Project\SDCS\Generative AI\Truck Simulink Model\TruckBenchmark_v1.2\TruckBenchmark\j1939.dbc
  J1939 Node Configuration3 : j1939protocollib/J1939 Node Configuration  Priority=-2  ConfigName=Config3  NodeID=Engine1  NodeName=Engine1  PrevNodeID=Custom  PrevConfig=Config  AllowAAC=off  NodeAddress=0  IndustryGroup=0  VehicleSystem=0  VehicleSystemInstance=0  FunctionID=0  FunctionInstance=0  ECUInstance=0  ManufacturerCode=0  IDNumber=0  SampleTime=-1  OutputAddress=off  OutputACStatus=off
  J1939 Transmit1 : j1939protocollib/J1939 Transmit  Priority=-1  ConfigName=Config2  NodeName=Engine1  PGList=CCVS(65265)  PGName=CCVS  MsgLength=8  SignalInfo=BrakeSwitch$28$2$1$2$1$0$1$0$0$3$$597$#ClutchSwitch$30$2$1$2$1$0$1$0$0$3$$598$#CruiseCtrlAccelerateSwitch$38$2$1$2$1$0$1$0$0$3$$602$#CruiseCtrlActive$24$2$1$2$1$0$1$0$0$3$$595$#CruiseCtrlCoastSwitch$34$2$1$2$1$0$1$0$0$3$$600$#CruiseCtrlEnableSwitch$26$2$1$2$1$0$1$0$0$3$$596$#CruiseCtrlPauseSwitch$4$2$1$2$1$0$1$0$0$3$$1633$#CruiseCtrlResumeSwitch$36$2$1$2$1$0$1$0$0$3$$601$#CruiseCtrlSetSpeed$40$8$1$2$1$0$1$0$0$250$km/h$86$#CruiseCtrlSetSwitch$32$2$1$2$1$0$1$0$0$3$$599$#CruiseCtrlStates$53$3$1$2$1$0$1$0$0$7$$527$#EngIdleDecrementSwitch$58$2$1$2$1$0$1$0$0$3$$967$#EngIdleIncrementSwitch$56$2$1$2$1$0$1$0$0$3$$968$#EngShutdownOverrideSwitch$62$2$1$2$1$0$1$0$0$3$$1237$#EngTestModeSwitch$60$2$1$2$1$0$1$0$0$3$$966$#PTOGovernorState$48$5$1$2$1$0$1$0$0$31$$976$#ParkBrakeReleaseInhibitRq$6$2$1$2$1$0$1$0$0$3$$3807$#ParkingBrakeSwitch$2$2$1$2$1$0$1$0$0$3$$70$#TwoSpeedAxleSwitch$0$2$1$2$1$0$1$0$0$3$$69$#WheelBasedVehicleSpeed$8$16$1$2$1$0$3.906250e-03$0$0$2.509960e+02$km/h$84$#  NSignals=20  StartBits=str2num('[double(28);double(30);double(38);double(24);double(34);double(26);double(4);double(36);double(40);double(32);double(53);double(58);double(56);double(62);double(60);double(48);double(6);double(2);double(0);double(8)]')  SignalSizes=str2num('[double(2),double(2),double(2),double(2),double(2),double(2),double(2),double(2),double(8),double(2),double(3),double(2),double(2),double(2),double(2),double(5),double(2),double(2),double(2),double(16)]')  ByteOrders=str2num('[int32(1);int32(1);int32(1);int32(1);int32(1);int32(1);int32(1);int32(1);int32(1);int32(1);int32(1);int32(1);int32(1);int32(1);int32(1);int32(1);int32(1);int32(1);int32(1);int32(1)]')  DataTypes=str2num('[int32(2);int32(2);int32(2);int32(2);int32(2);int32(2);int32(2);int32(2);int32(2);int32(2);int32(2);int32(2);int32(2);int32(2);int32(2);int32(2);int32(2);int32(2);int32(2);int32(2)]')  MultiplexTypes=str2num('[int32(1);int32(1);int32(1);int32(1);int32(1);int32(1);int32(1);int32(1);int32(1);int32(1);int32(1);int32(1);int32(1);int32(1);int32(1);int32(1);int32(1);int32(1);int32(1);int32(1)]')  MultiplexValues=str2num('[double(0);double(0);double(0);double(0);double(0);double(0);double(0);double(0);double(0);double(0);double(0);double(0);double(0);double(0);double(0);double(0);double(0);double(0);double(0);double(0)]')  Factors=str2num('[double(1);double(1);double(1);double(1);double(1);double(1);double(1);double(1);double(1);double(1);double(1);double(1);double(1);double(1);double(1);double(1);double(1);double(1);double(1);double(3.906250e-03)]')  Offsets=str2num('[double(0);double(0);double(0);double(0);double(0);double(0);double(0);double(0);double(0);double(0);double(0);double(0);double(0);double(0);double(0);double(0);double(0);double(0);double(0);double(0)]')  Minimums=str2num('[double(0);double(0);double(0);double(0);double(0);double(0);double(0);double(0);double(0);double(0);double(0);double(0);double(0);double(0);double(0);double(0);double(0);double(0);double(0);double(0)]')  Maximums=str2num('[double(3);double(3);double(3);double(3);double(3);double(3);double(3);double(3);double(250);double(3);double(7);double(3);double(3);double(3);double(3);double(31);double(3);double(3);double(3);double(2.509960e+02)]')  Units=0  SPN=str2num('[double(597);double(598);double(602);double(595);double(600);double(596);double(1633);double(601);double(86);double(599);double(527);double(967);double(968);double(1237);double(966);double(976);double(3807);double(70);double(69);double(84)]')  Comment=0  PGPriority=6  DestAddrID=Custom  DestAddrName=255  TransmitPeriodically=on  MessagePeriod=0  SampleTime=-1  ApplyMinMax=off
  Signals4 : Scope  NumInputPorts=4
  To Workspace : ToWorkspace  VariableName=canraw65265  SaveFormat=Timeseries  SampleTime=-1
      settings: Save2DSignal=2-D array (concatenate along first dimension)
  wires:
  Data Type Conversion5/1 -> J1939 Transmit1/4, CAN Pack/4
  Data Type Conversion19/1 -> CAN Pack/19, J1939 Transmit1/19
  Constant29/1 -> Data Type Conversion10/1
  Velocity/1 -> Signals4/4, J1939 Transmit1/20, CAN Pack/20
  Data Type Conversion15/1 -> CAN Pack/15, J1939 Transmit1/15
  Data Type Conversion7/1 -> CAN Pack/6, J1939 Transmit1/6
  Clutch Pos/1 -> Signals4/2, CAN Pack/2, J1939 Transmit1/2
  Data Type Conversion14/1 -> CAN Pack/14, J1939 Transmit1/14
  Data Type Conversion13/1 -> CAN Pack/13, J1939 Transmit1/13
  Constant36/1 -> Data Type Conversion7/1
  trigger/1 -> J1939 Transmit1/21  "Trigger"
  Constant34/1 -> Data Type Conversion5/1
  Data Type Conversion1/1 -> CAN Pack/1, J1939 Transmit1/1
  Data Type Conversion18/1 -> CAN Pack/18, J1939 Transmit1/18
  Data Type Conversion17/1 -> CAN Pack/17, J1939 Transmit1/17
  Data Type Conversion12/1 -> CAN Pack/12, J1939 Transmit1/12
  Data Type Conversion6/1 -> CAN Pack/5, J1939 Transmit1/5
  Constant24/1 -> Data Type Conversion15/1
  Constant21/1 -> Data Type Conversion11/1
  Constant27/1 -> Data Type Conversion18/1
  Constant22/1 -> Data Type Conversion12/1
  Constant38/1 -> Data Type Conversion9/1
  Constant33/1 -> Data Type Conversion4/1
  Data Type Conversion21/1 -> Signals4/3, CAN Pack/9, J1939 Transmit1/9
  Constant30/1 -> Data Type Conversion1/1
  Constant26/1 -> Data Type Conversion17/1
  Constant35/1 -> Data Type Conversion6/1
  Data Type Conversion8/1 -> CAN Pack/7, J1939 Transmit1/7
  Gain1/1 -> Data Type Conversion21/1
  Constant39/1 -> Gain1/1
  Constant32/1 -> Data Type Conversion13/1
  Constant25/1 -> Data Type Conversion16/1
  CAN Pack/1 -> To Workspace/1
  Constant37/1 -> Data Type Conversion8/1
  Data Type Conversion16/1 -> CAN Pack/16, Signals4/1, J1939 Transmit1/16
  Data Type Conversion9/1 -> CAN Pack/8, J1939 Transmit1/8
  Data Type Conversion10/1 -> CAN Pack/10, J1939 Transmit1/10
  Constant28/1 -> Data Type Conversion19/1
  Data Type Conversion4/1 -> CAN Pack/3, J1939 Transmit1/3
  Constant23/1 -> Data Type Conversion14/1
  Data Type Conversion11/1 -> CAN Pack/11, J1939 Transmit1/11

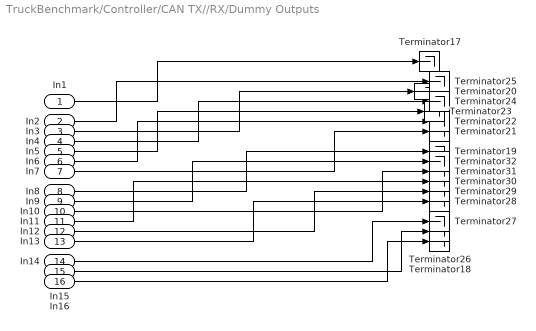
== system TruckBenchmark/Controller/CAN TX//RX/Dummy Outputs ==
  In1 : Inport
  In2 : Inport  Port=2
  In3 : Inport  Port=3
  In4 : Inport  Port=4
  In5 : Inport  Port=5
  In6 : Inport  Port=6
  In7 : Inport  Port=7
  In8 : Inport  Port=8
  In9 : Inport  Port=9
  In10 : Inport  Port=10
  In11 : Inport  Port=11
  In12 : Inport  Port=12
  In13 : Inport  Port=13
  In14 : Inport  Port=14
  In15 : Inport  Port=15
  In16 : Inport  Port=16
  Terminator{17..32} (16 alike) : Terminator
  wires:
  In14/1 -> Terminator27/1
  In6/1 -> Terminator22/1
  In5/1 -> Terminator23/1
  In7/1 -> Terminator21/1
  In9/1 -> Terminator32/1
  In15/1 -> Terminator26/1
  In4/1 -> Terminator24/1
  In11/1 -> Terminator30/1
  In1/1 -> Terminator17/1
  In3/1 -> Terminator20/1
  In13/1 -> Terminator28/1
  In12/1 -> Terminator29/1
  In16/1 -> Terminator18/1
  In10/1 -> Terminator31/1
  In2/1 -> Terminator25/1
  In8/1 -> Terminator19/1

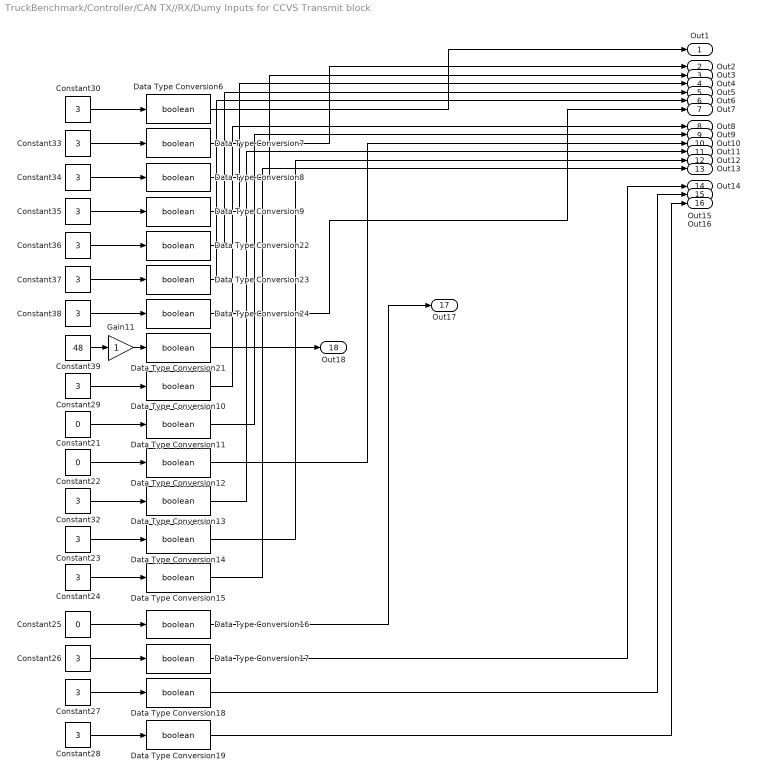
== system TruckBenchmark/Controller/CAN TX//RX/Dumy Inputs for CCVS Transmit block ==
  Constant21 : Constant  Value=0
  Constant22 : Constant  Value=0
  Constant{23..24,26..30,32..38} (14 alike) : Constant  Value=3
  Constant25 : Constant  Value=0
  Constant39 : Constant  Value=48
  Data Type Conversion{6..19,21..24} (18 alike) : DataTypeConversion  OutDataTypeStr=boolean  SaturateOnIntegerOverflow=off  RndMeth=Floor
  Gain11 : Gain
  Out1 : Outport
  Out2 : Outport  Port=2
  Out3 : Outport  Port=3
  Out4 : Outport  Port=4
  Out5 : Outport  Port=5
  Out6 : Outport  Port=6
  Out7 : Outport  Port=7
  Out8 : Outport  Port=8
  Out9 : Outport  Port=9
  Out10 : Outport  Port=10
  Out11 : Outport  Port=11
  Out12 : Outport  Port=12
  Out13 : Outport  Port=13
  Out14 : Outport  Port=14
  Out15 : Outport  Port=15
  Out16 : Outport  Port=16
  Out17 : Outport  Port=17
  Out18 : Outport  Port=18
  wires:
  Constant39/1 -> Gain11/1
  Data Type Conversion21/1 -> Out18/1
  Constant21/1 -> Data Type Conversion11/1
  Constant26/1 -> Data Type Conversion17/1
  Data Type Conversion11/1 -> Out9/1
  Constant32/1 -> Data Type Conversion13/1
  Data Type Conversion16/1 -> Out17/1
  Constant28/1 -> Data Type Conversion19/1
  Data Type Conversion8/1 -> Out3/1
  Data Type Conversion13/1 -> Out11/1
  Data Type Conversion19/1 -> Out16/1
  Data Type Conversion6/1 -> Out1/1
  Data Type Conversion14/1 -> Out12/1
  Data Type Conversion17/1 -> Out14/1
  Data Type Conversion9/1 -> Out4/1
  Constant33/1 -> Data Type Conversion7/1
  Constant30/1 -> Data Type Conversion6/1
  Constant23/1 -> Data Type Conversion14/1
  Gain11/1 -> Data Type Conversion21/1
  Constant37/1 -> Data Type Conversion23/1
  Data Type Conversion12/1 -> Out10/1
  Constant35/1 -> Data Type Conversion9/1
  Constant25/1 -> Data Type Conversion16/1
  Constant29/1 -> Data Type Conversion10/1
  Data Type Conversion15/1 -> Out13/1
  Data Type Conversion22/1 -> Out5/1
  Constant24/1 -> Data Type Conversion15/1
  Data Type Conversion10/1 -> Out8/1
  Data Type Conversion7/1 -> Out2/1
  Constant34/1 -> Data Type Conversion8/1
  Constant27/1 -> Data Type Conversion18/1
  Constant38/1 -> Data Type Conversion24/1
  Constant22/1 -> Data Type Conversion12/1
  Constant36/1 -> Data Type Conversion22/1
  Data Type Conversion24/1 -> Out7/1
  Data Type Conversion23/1 -> Out6/1
  Data Type Conversion18/1 -> Out15/1

== system TruckBenchmark/Controller/CAN TX//RX/J1939 CAN Transport Layer1 ==
  CAN Configuration : S-Function  LoadFcn=set_param(gcb, 'BlockHandle', num2str(gcbh));  FunctionName=svntcanconfig  Parameters=BlockHandle, Device, ObjConstructor, BusSpeed, EnableBitParameters, SJW, TSEG1, TSEG2, NSamples, AckMode  SFunctionDeploymentMode=off  EnableBusSupport=off  mask(CAN Configuration){BlockHandle=825.0001, Device=MathWorks Virtual 1 (Channel 1), ObjConstructor=canChannel('MathWorks', 'Virtual 1', 1), BusSpeed=250000, EnableBitParameters=off, SJW=1, TSEG1=4, TSEG2=3, NSamples=1, AckMode=Normal}
      mask prompts: BlockHandle "Block handle"; Device "Device Name"; ObjConstructor "Object constructor"; BusSpeed "Bus speed:"; EnableBitParameters "Set bit parameters manually"; SJW "Synchronization jump width (SJW):"; TSEG1 "Time segment 1 (TSEG1)"; TSEG2 "Time segment 2 (TSEG2)"; NSamples "Number of samples:"; AckMode "Acknowledge mode:"
      mask help: Configure the properties for the specified CAN device.
      mask Help: eval('helpview(fullfile(docroot, ''toolbox'', ''vnt'', ''vnt.map''), ''vnt_canconfig_block'')');
      mask TypeOptions AckMode: Normal | Silent
  CAN Receive : S-Function  LoadFcn=set_param(gcb, 'BlockHandle', num2str(gcbh));  FunctionName=svntcanreceive  Parameters=BlockHandle, Device, ObjConstructor, EnableStandardIDsFilter, StandardIDs, EnableExtendedIDsFilter, ExtendedIDs, SampleTime, MsgsPerTimestep, StdIDsCombo, ExtIDsCombo, InternalFilterUpdateStatus, BusOutput  SFunctionDeploymentMode=off  EnableBusSupport=off  mask(CAN Receive){BlockHandle=826.0004, Device=MathWorks Virtual 1 (Channel 1), ObjConstructor=canChannel('MathWorks', 'Virtual 1', 1), EnableStandardIDsFilter=off, StandardIDs=0, EnableExtendedIDsFilter=off, ExtendedIDs=0, SampleTime=can_sample_time, MsgsPerTimestep=all, StdIDsCombo=Allow all, ExtIDsCombo=Allow all, InternalFilterUpdateStatus=on, BusOutput=off}
      mask prompts: BlockHandle "Block handle"; Device "Device Name"; ObjConstructor "Object constructor"; EnableStandardIDsFilter "Filter for accepted Standard ID range"; StandardIDs "Standard IDs"; EnableExtendedIDsFilter "Filter for accepted Extended ID range"; ExtendedIDs "Extended IDs"; SampleTime "Sample time:"; MsgsPerTimestep "Messages per timestep"; StdIDsCombo "Standard IDs Combo"; ExtIDsCombo "Extended IDs Combo"; InternalFilterUpdateStatus "Internal Filter update"; BusOutput "Output as bus"
      mask help: Receive CAN Messages using the specified CAN device.
      mask Help: eval('helpview(fullfile(docroot, ''toolbox'', ''vnt'', ''vnt.map''), ''vnt_canrec_block'')');
      mask TypeOptions MsgsPerTimestep: 1 | all
      mask TypeOptions StdIDsCombo: Allow all | Allow only | Block only
      mask TypeOptions ExtIDsCombo: Allow all | Allow only | Block only
  CAN Transmit Subsystem : Subsystem  TreatAsAtomicUnit=on
  Data Type Conversion : DataTypeConversion  Commented=on  SaturateOnIntegerOverflow=off  RndMeth=Floor
  J1939 Transport Layer Transmit : S-Function  FunctionName=slcantx  Parameters=TLID, TLTag, MaxNumMessages, SampleTime  SFunctionDeploymentMode=off  EnableBusSupport=off  mask(J1939 Transport Layer Transmit){TLID=Config1, MaxNumMessages=20, SampleTime=can_sample_time}
      mask prompts: TLID "Config ID:"; MaxNumMessages "Maximum number of messages:"; SampleTime "Sample time:"
      mask help:
      | Processes the queued J1939 messages and sends to the
      | protocol (CAN) transmit block for transmission.
      mask init:
      | [str, port] = j1939.internal.getTLDisplayString;
      | TLTag = j1939.internal.getTLParams;
      mask Help: uiwait(warndlg('Yet to be tagged'));
      mask Display:
      | disp(str);
      | port_label('output',port(1).id,port(1).label);
      | port_label('output',port(2).id,port(2).label);
  J1939 Transport Layer Receive Subsystem : Subsystem  TreatAsAtomicUnit=on
  To Workspace : ToWorkspace  Commented=on  VariableName=can_raw_data  SaveFormat=Timeseries  SampleTime=-1
      settings: Save2DSignal=2-D array (concatenate along first dimension)
  wires:
  J1939 Transport Layer Transmit/1 -> Data Type Conversion/1, CAN Transmit Subsystem/1(CAN Msg)
  J1939 Transport Layer Transmit/2 -> CAN Transmit Subsystem/2(N)
  CAN Receive/2 -> J1939 Transport Layer Receive Subsystem/1(In1)
  CAN Receive/1 -> J1939 Transport Layer Receive Subsystem/Trigger
  Data Type Conversion/1 -> To Workspace/1
